simulink model "acausalFiltering_t5"  (R2012b)
settings: Solver=FixedStepDiscrete  StartTime=0.0  StopTime=10.0  FixedStep=0.001  RelTol=1e-3
undefined symbols (not defined in the file): dfilt
libraries: dsparch4 x2
settings Model: BufferReuse=off  Creator=gilja  LastModifiedBy=NPTL
settings SolverCC: EnableConcurrentExecution=on  ConcurrentTasks=on
settings DataIOCC: SaveOutput=off  SignalLogging=off  DSMLogging=off  SaveTime=off
settings OptimizationCC: InlineParams=on  InlineInvariantSignals=on  OptimizeBlockIOStorage=off  BufferReuse=off  ExpressionFolding=off  LocalBlockOutputs=off
settings HardwareCC: ProdIntDivRoundTo=Zero  ProdEndianess=LittleEndian  ProdHWDeviceType=Generic->32-bit x86 compatible
settings ModelReferenceCC: ModelReferenceMinAlgLoopOccurrences=on
settings RTWCC: SystemTargetFile=xpctarget.tlc  TemplateMakefile=xpc_default_tmf  Description=xPC Target  ProcessScript=xpctarget_make_rtw_hook  RTWCompilerOptimization=On
settings CodeAppCC: MaxIdLength=62
settings xpcTargetCC: TargetFcnLib=ansi_tfl_table_tmw.mat  CodeReplacementLibrary=XPC_BLAS  ParMdlRefBuildCompliant=on  ConcurrentExecutionCompliant=on  CombineSignalStateStructs=off  GRTInterface=on  xPCTaskExecutionProfile=on  xPCRL32EventNumber=5000  xPCisDownloadable=off  xPCLoadParamSetFile=off  xPCConcurrentTasks=off  xPCEnableSFAnimation=off

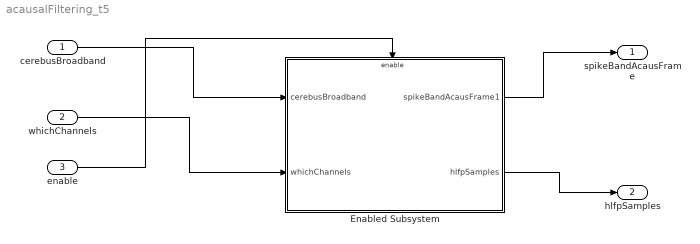
== system acausalFiltering_t5 ==
  cerebusBroadband : Inport  OutDataTypeStr=Bus: cerebusBroadband
  whichChannels : Inport  Port=2  PortDimensions=[1 32]
  enable : Inport  Port=3  OutDataTypeStr=uint8  PortDimensions=[1 1]
  Enabled Subsystem : Subsystem  TreatAsAtomicUnit=on
  spikeBandAcausFrame : Outport  BusOutputAsStruct=on
  hlfpSamples : Outport  Port=2  BusOutputAsStruct=on
  wires:
  cerebusBroadband/1 -> Enabled Subsystem/1(cerebusBroadband)
  whichChannels/1 -> Enabled Subsystem/2(whichChannels)
  enable/1 -> Enabled Subsystem/Enable
  Enabled Subsystem/1(spikeBandAcausFrame1) -> spikeBandAcausFrame/1
  Enabled Subsystem/2(hlfpSamples) -> hlfpSamples/1

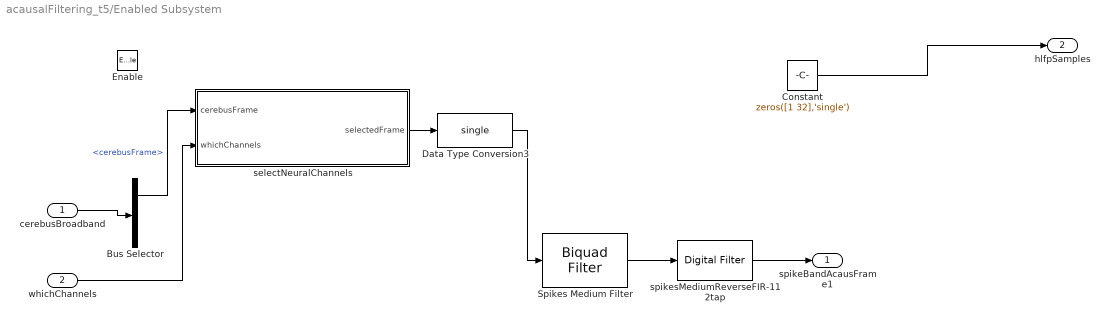
== system acausalFiltering_t5/Enabled Subsystem ==
  cerebusBroadband : Inport  OutDataTypeStr=Bus: cerebusBroadband
  whichChannels : Inport  Port=2  PortDimensions=[1 32]
  Enable : EnablePort
  Bus Selector : BusSelector  OutputSignals=cerebusFrame,outputValid
  Constant : Constant  Value=zeros([1 32],'single')
  Data Type Conversion3 : DataTypeConversion  OutDataTypeStr=single
  Spikes Medium Filter : dsparch4/Biquad Filter  IIRFiltStruct=Direct form II transposed  CoeffSource=Specify via dialog  BiQuadCoeffs="[0.95321773445431  -1.90644870937033 0.95323097500802 1 -1.90514144409761 0.90775595733389;  0.97970016700443  -1.95938672569874 0.97968655878878 1 -1.95804317832840 0.96073029104793]"  a0Flag=Warning  IC=0  ICnum=0  ICden=0  InputProcessing=Columns as channels (frame based)  denAccumFracLength=30  denProdOutputFracLength=30  secondMemoryFracLength=15  roundingMode=Floor  overflowMode=off  ScaleValues=1  optimizeScaleValues=on  ScaleValueMode=Specify via input port (g)  scaleValueFracLength=14  FilterSource=Specify via dialog  dfiltObjectName=dfilt.df2tsos([1 0.3 0.4],[1 0.1 0.2])
  selectNeuralChannels : MATLAB Function  TreatAsAtomicUnit=on
  spikesMediumReverseFIR-112tap : dsparch4/Digital Filter  Tag=BlockMethodSubSystem  TypePopup=FIR (all zeros)  IIRFiltStruct=Direct form II transposed  AllPoleFiltStruct=Direct form  FIRFiltStruct=Direct form  CoeffSource=Specify via dialog  NumCoeffs=[-0.00496114643282997 -0.00511944203138304 -0.00526878677381715 -0.00540837410973427 -0.00553739273290177 -0.00565502881313373 -0.00576046833931565 -0.00585289957239577 -0.00593151560680727 -0.00599551703852563 -0.00604411473759436 -0.00607653272264253 -0.00609201113457714 -0.00608980930630343 -0.00606920892497043 -0.00602951728290735 -0.00597007061307309 -0.00589023750448747 -0.00578942239278268 -0.00566706912066117 -0.00552266456273154 -0.00535574230882618 -0.00516588639961058 -0.0049527351079659 -0.00471598475930157 -0.00445539358366996 -0.00417078559226303 -0.00386205447057114 -0.00352916748025151 -0.00317216936147669 -0.00279118622730723 -0.00238642944142276 -0.00195819947033915 -0.00150688970105406 -0.00103299021493475 -0.000537091508489796 -1.98881515925963e-05 0.000517817626386806 0.00107511243212321 0.00165096829517208 0.00224423935571616 0.00285365866281217 0.00347783509266308 0.00411525039633964 0.0047642563862732 0.00542307227062888 0.00608978214453903 0.00676233264686876 0.00743853079099066 0.00811604197766102 0.00879238819781258 0.00946494643265294 0.0101309472580707 0.0107874736598251 0.011431460065609 0.0120596915994152 0.0126688035631636 0.0132552811498886 0.0138154593921088 0.0143455233484383 0.0148415085306105 0.0152993015724897 0.0157146411418049 0.0160831190944893 0.0164001818707454 0.0166611321310562 0.0168611306294592 0.0169951983205324 0.0170582186955749 0.0170449403425982 0.016949979723638 0.0167678241621559 0.0164928350321601 0.016119251139786 0.0156411922871306 0.0150526630071707 0.0143475564576735 0.0135196584610761 0.0125626516765248 0.0114701198892456 0.0102355524018378 0.00885234851109312 0.00731382205342658 0.00561320600126308 0.00374365709216062 0.00169826047200783 -0.000529965666824618 -0.00294806547178339 -0.00556314086048071 -0.00838234701481222 -0.0114128879584571 -0.0146620122372828 -0.0181370087217753 -0.0218452025501726 -0.0257939512302837 -0.0299906409172236 -0.034442682883063 -0.0391575101934262 -0.0441425746042988 -0.049405343690809 -0.0549532982176949 -0.0607939297589152 -0.0669347385714719 -0.0733832317254782 -0.0801469214896301 -0.0872333239676136 -0.094649957977231 -0.102404344159842 -0.110504004303203 -0.118956460855762 -0.127769236605171 0.933865781722487]  DenCoeffs=[1 0.1]  BiQuadCoeffs=[1 0.3 0.4 1 0.1 0.2]  LatticeCoeffs=[0.2 0.4]  denIgnore=on  FiltPerSampPopup=One filter per frame  IC=0  ICnum=0  ICden=0  roundingMode=Floor  overflowMode=off  ScaleValues=1  scaleValueFracLength=14  stageInFracLength=15  stageOutFracLength=15  FilterSource=Specify via dialog  dfiltObjectName=dfilt.dffir([1 2 1])  InputProcessing=Columns as channels (frame based)
  spikeBandAcausFrame1 : Outport  BusOutputAsStruct=on
  hlfpSamples : Outport  Port=2  BusOutputAsStruct=on
  wires:
  spikesMediumReverseFIR-112tap/1 -> spikeBandAcausFrame1/1
  cerebusBroadband/1 -> Bus Selector/1
  Data Type Conversion3/1 -> Spikes Medium Filter/1
  Spikes Medium Filter/1 -> spikesMediumReverseFIR-112tap/1
  whichChannels/1 -> selectNeuralChannels/2(whichChannels)
  Bus Selector/1 -> selectNeuralChannels/1(cerebusFrame)  "<cerebusFrame>"
  selectNeuralChannels/1(selectedFrame) -> Data Type Conversion3/1
  Constant/1 -> hlfpSamples/1

== matlab function acausalFiltering_t5/Enabled Subsystem/selectNeuralChannels ==
  data: cerebusFrame input; whichChannels input double size=[1 32]; selectedFrame output
function selectedFrame = selectNeuralChannels(cerebusFrame, whichChannels)
%#codegen
persistent selectedFrameTmp
if(isempty(selectedFrameTmp))
    selectedFrameTmp = zeros(size(cerebusFrame, 1), 32);
end

selectedFrameTmp(:,1:32) = cerebusFrame(:,whichChannels);

selectedFrame = selectedFrameTmp;
